simulink model "Demo_PreScanCarSim3D_cs"  (Simulink 7.6)
settings: Solver=ode5  SolverMode=SingleTasking  StartTime=0.0  StopTime=68  FixedStep=1/400  RelTol=1e-3
PreLoadFcn:
  | check_NUTS_defined;
  | 
  | assignin('base',['model_closed_' bdroot],false);
InitFcn:
  | PreScanExperimentInitFcn(bdroot)
StopFcn:
  | PreScanExperimentStopFcn(bdroot)
undefined symbols (not defined in the file or in its folder): DiscIntNeverNeededParam, warningInitialVelocity, x0, x_ini_VRML, y_ini_VRML, z_ini_VRML
libraries: PreScanSimulinkLibrary x13, simulink_extras x5, PreScanUsefulBlocks x5, simulink x3, Solver_SF x1
(part 5 of 10)

== system Demo_PreScanCarSim3D_cs/Audi_A8_1/CarSim_Vehicle ==
  note: Source model: .\CarSim_Data\Extensions\Simulink\CarSim_VehicleDynamics.mdl
  note: For state mode 'Dynamic' positions
      | are not taken into account, as they
      | are computed by integrating velocity.
      | Click annotation for Help.
  PathFollower_In : Inport
  Contact_In : Inport  Port=2
  CarSim S-Function : Solver_SF/CarSim S-Function  Priority=1  VehicleCode=i_i  SIMFILE=./CarSim_Data/simfile.sim
  CarSim2PreScanSTATE : Subsystem  mask(CarSim2PreScan:){z0=0.241}
      mask prompts: z0 "PreScan Actor initial COG z-position wrt GLOBAL axis system [m]"
      mask help: This block converts the outputs coming from the CarSim block into consistent PreScan signals.
  CarSim2PreScan_BUS : Subsystem  mask(PreScan block: CarSim to PreScan BUS){TyreRadius=0.358, cogZOffset=0.241}
      mask prompts: TyreRadius "Tyre Radius [m]"; cogZOffset "cog Z offset [m]"
      mask help: CarSim to PreScan BUS selector
      mask Help: eval('openHelp()')
      mask Display: disp('PreScan BUS\nVehicleDynamics')
  CarSim2PreScan_ContactAdapter : Subsystem  Tag=CarSim2PreScan_ContactAdapter  mask{wheelRadius=0.358}
      mask prompts: wheelRadius "Wheel radius:"
  Demux2 : Demux  Outputs=3
  Mux : Mux  Inputs=[1 1 1 12]
  MuxState : Subsystem  Tag=MuxState  mask{positioningmode=on, TimeStep=1/400}
      mask prompts: positioningmode "Positioning Mode"; TimeStep "Auto Assigned: Time Step [s]"
      settings: DeleteFcn=PreScanBlockDeleteFcn;
  TyreContact To Road Information : Subsystem  mask{Roll0=0, Pitch0=0, Yaw0=0.029771632590382069}
      mask prompts: Roll0 "Ini roll-angle BODY wrt VEHICLE axis system [deg]"; Pitch0 "Ini pitch-angle BODY wrt VEHICLE axis system [deg]"; Yaw0 "Ini yaw-angle VEHICLE wrt GLOBAL axis system [deg]"
  State : Outport
  State_BUS : Outport  Port=2
  ContactParams : Outport  Port=3
  wires:
  Mux/1 -> CarSim S-Function/1
  Demux2/1 -> Mux/1
  Demux2/2 -> Mux/2
  Demux2/3 -> Mux/3
  PathFollower_In/1 -> Demux2/1
  TyreContact To Road Information/1(RoadSlopeAndZ_[FL;FR;RL;RR]) -> Mux/4
  CarSim2PreScan_BUS/1(PreScanBUS_VehicleDynamics) -> State_BUS/1, CarSim2PreScan_ContactAdapter/2(State_Bus)
  CarSim S-Function/1 -> CarSim2PreScanSTATE/1(CarSim_In), CarSim2PreScan_BUS/1(CarSim_In)
  Contact_In/1 -> TyreContact To Road Information/1(TyreInfo_in)
  MuxState/1(state) -> State/1, CarSim2PreScan_ContactAdapter/1(State)
  CarSim2PreScan_ContactAdapter/1(ContactParams) -> ContactParams/1
  CarSim2PreScanSTATE/9(Y [rad]) -> MuxState/9(Y [rad])
  CarSim2PreScanSTATE/8(P [rad]) -> MuxState/8(P [rad])
  CarSim2PreScanSTATE/7(R [rad]) -> MuxState/7(R [rad])
  CarSim2PreScanSTATE/6(dz [m/s]) -> MuxState/6(dz [m/s])
  CarSim2PreScanSTATE/5(dy [m/s]) -> MuxState/5(dy [m/s])
  CarSim2PreScanSTATE/4(dx [m/s]) -> MuxState/4(dx [m/s])
  CarSim2PreScanSTATE/3(z [m]) -> MuxState/3(z [m])
  CarSim2PreScanSTATE/2(y [m]) -> MuxState/2(y [m])
  CarSim2PreScanSTATE/1(x [m]) -> MuxState/1(x [m])

== system Demo_PreScanCarSim3D_cs/Audi_A8_1/PathFollower_Preview_1 ==
  TrajOffset x,y,Y [m,m,deg] : Inport
  ActorOffset_Left(+) / Right(-) [m] : Inport  Port=2
  position x,y,Y [m,m,deg] : Inport  Port=3
  Initial Velocity [m/s] : Inport  Port=4
  Desired Velocity [m/s] : Inport  Port=5
  velocity [m/s] : Inport  Port=6
  vx [m/s] : Inport  Port=7
  vy [m/s] : Inport  Port=8
  Yaw rate [deg/s] : Inport  Port=9
  CorneringStiffness_Tyres_Front [N/rad] : Inport  Port=10
  CorneringStiffness_Tyres_Rear [N/rad] : Inport  Port=11
  steering_ratio[-] : Inport  Port=12
  LateralController : Subsystem
  LongitudinalController : Subsystem
  delta_steerwheel [deg] : Outport
  throttle [%] : Outport  Port=2
  brake pressure [bar] : Outport  Port=3
  v0 [m/s] : Outport  Port=4
  Auto_GearShift : Outport  Port=5
  Actor/Traj_distance [m] : Outport  Port=6
  Actor/Traj_angle [deg] : Outport  Port=7
  wires:
  LateralController/3(delta_steerwheel [deg]) -> delta_steerwheel [deg]/1
  steering_ratio[-]/1 -> LateralController/9(steering_ratio[-])
  CorneringStiffness_Tyres_Rear [N/rad]/1 -> LateralController/8(CorneringStiffness_Tyres_Rear [N/rad])
  CorneringStiffness_Tyres_Front [N/rad]/1 -> LateralController/7(CorneringStiffness_Tyres_Front [N/rad])
  Yaw rate [deg/s]/1 -> LateralController/6(Yaw rate [deg/s])
  vy [m/s]/1 -> LateralController/5(vy [m/s])
  vx [m/s]/1 -> LateralController/4(vx [m/s])
  position x,y,Y [m,m,deg]/1 -> LateralController/3(position x,y,Y [m,m,deg])
  ActorOffset_Left(+) / Right(-) [m]/1 -> LateralController/2(ActorOffset_Left(+) / Right(-) [m])
  TrajOffset x,y,Y [m,m,deg]/1 -> LateralController/1(TrajOffset x,y,Y [m,m,deg])
  LateralController/2(Actor/Traj_angle [deg]) -> Actor/Traj_angle [deg]/1
  LateralController/1(Actor/Traj_distance [m]) -> Actor/Traj_distance [m]/1
  velocity [m/s]/1 -> LongitudinalController/1(v_actual [m/s])
  LongitudinalController/1(throttle [%]) -> throttle [%]/1
  Desired Velocity [m/s]/1 -> LongitudinalController/2(Desired Velocity [m/s])
  Initial Velocity [m/s]/1 -> LongitudinalController/3(Initial Velocity [m/s])
  LongitudinalController/2(brake pressure [bar]) -> brake pressure [bar]/1
  LongitudinalController/3(v0 [m/s]) -> v0 [m/s]/1
  LongitudinalController/4(Auto_GearShift) -> Auto_GearShift/1

== system Demo_PreScanCarSim3D_cs/Audi_A8_1/PreScan_RayCast_Contact_Sensor ==
  ContactParams : Inport  SampleTime=TimeStep
  Bus Creator2 : BusCreator
  Constant : Constant  Value=0
  Contact Point Bus Creator : Subsystem
  Contact Point Bus Creator1 : Subsystem
  Contact Point Bus Creator2 : Subsystem
  Contact Point Bus Creator3 : Subsystem
  Demux : Demux
  Demux1 : Demux  Outputs=[9 1 12 4]
  Demux2 : Demux
  Level-2 M-file S-Function : M-S-Function  FunctionName=msfcn_wheelPoseCorrection  Parameters=nrOfWheels  mask{nrOfWheels=4}
      mask prompts: nrOfWheels "Number of Wheels:"
      mask Display:
      | port_label('input', 1,'Wheel poses')
      | port_label('input', 2,'Wheel radius')
      | port_label('input', 3,'Vehicle orientation')
      | 
      | port_label('output', 1,'Virtual poses')
  Level-2 MATLAB S-Function : M-S-Function  FunctionName=msfcn_wheelContacts_raycast  Parameters=NumberOfWheels, MaxContactPoints, Range  mask{NumberOfWheels=4, MaxContactPoints=1, Range=4}
      mask prompts: NumberOfWheels "Number of Wheels:"; MaxContactPoints "Maximum number of Contact Points:"; Range "Range of ray [m]:"
      mask Display:
      | port_label('input', 1, 'Wheel poses')
      | 
      | port_label('output', 1, 'Contacts')
  Level-2 MATLAB S-Function1 : M-S-Function  FunctionName=msfcn_CollisionConv  Parameters=NumberOfWheels hcog b  mask{NumberOfWheels=4}
      mask prompts: NumberOfWheels "Number of Wheels:"
      settings: AttributesFormatString=Wheels = %<NumberOfWheels>
      mask Display:
      | port_label('input', 1,'Vehicle wrt World')
      | port_label('input', 2,'Wheels wrt World')
  Mux6 : Mux  Inputs=2
  Rate Transition : RateTransition  OutPortSampleTimeOpt=Inherit
  Vehicle Local to World : Subsystem
  Wheels Local to World : Subsystem  Tag=MuxWheels
      settings: DeleteFcn=PreScanBlockDeleteFcn;
      mask Type: PreScan Mux Block:
  Results : Outport
  wires:
  Rate Transition/1 -> Results/1
  Demux1/4 -> Level-2 M-file S-Function/2
  Level-2 M-file S-Function/1 -> Level-2 MATLAB S-Function/1
  Level-2 MATLAB S-Function1/1 -> Level-2 M-file S-Function/1
  Mux6/1 -> Level-2 MATLAB S-Function1/1
  Level-2 MATLAB S-Function/1 -> Demux/1
  Demux/1 -> Contact Point Bus Creator/1(demux in)
  Demux/2 -> Contact Point Bus Creator1/1(demux in)
  Demux/3 -> Contact Point Bus Creator2/1(demux in)
  Demux/4 -> Contact Point Bus Creator3/1(demux in)
  Contact Point Bus Creator/1(bus out) -> Bus Creator2/1  "TireFL"
  Contact Point Bus Creator1/1(bus out) -> Bus Creator2/2  "TireFR"
  Contact Point Bus Creator2/1(bus out) -> Bus Creator2/3  "TireRL"
  Contact Point Bus Creator3/1(bus out) -> Bus Creator2/4  "TireRR"
  Vehicle Local to World/1(Position) -> Mux6/1
  Vehicle Local to World/2(Orientation) -> Level-2 M-file S-Function/3, Mux6/2
  Wheels Local to World/1(Wheel Poses) -> Level-2 MATLAB S-Function1/2
  Demux1/2 -> Wheels Local to World/3(Velocity [m/s])
  Demux2/1 -> Wheels Local to World/4(Disp FL [m])
  Demux2/2 -> Wheels Local to World/5(Disp FR [m])
  Demux2/3 -> Wheels Local to World/6(Disp RL [m])
  Demux2/4 -> Wheels Local to World/7(Disp RR [m])
  Constant/1 -> Wheels Local to World/2(Steer Angle Rear [deg]), Wheels Local to World/1(Steer Angle Front [deg])
  Bus Creator2/1 -> Rate Transition/1
  ContactParams/1 -> Demux1/1
  Demux1/1 -> Vehicle Local to World/1(State)
  Demux1/3 -> Demux2/1

== system Demo_PreScanCarSim3D_cs/Audi_A8_1/SELF_Demux ==
  SELF : Inport
  Demux1 : Demux  Outputs=3
  Demux2 : Demux  Outputs=3
  Demux3 : Demux  Outputs=[3 3 1 1]
  Demux4 : Demux  Outputs=3
  Gain : Gain  Gain=180/pi
  Gain1 : Gain  Gain=180/pi
  Selector : Selector  InputPortWidth=3  IndexOptions=Index vector (dialog)  Indices=[3]  OutputSizes=1
  compas converter : Subsystem
  xyz2GPS : PreScanUsefulBlocks/xyz2GPS  CoordinateCount=1  GPS_base=[0.000000 0.000000 0.000]
  x [m] : Outport
  y [m] : Outport  Port=2
  z [m] : Outport  Port=3
  rotx [deg] : Outport  Port=4
  roty [deg] : Outport  Port=5
  rotz [deg] : Outport  Port=6
  GPS lat [deg] : Outport  Port=7
  GPS long [deg] : Outport  Port=8
  GPS alt [m] : Outport  Port=9
  velocity [m/s] : Outport  Port=10
  heading [deg] : Outport  Port=11
  yaw rate [deg/s] : Outport  Port=12
  wires:
  Demux3/4 -> Gain1/1
  Gain1/1 -> yaw rate [deg/s]/1
  Demux3/3 -> velocity [m/s]/1
  compas converter/1(heading [deg]) -> heading [deg]/1
  xyz2GPS/1 -> Demux4/1
  Demux4/3 -> GPS alt [m]/1
  Demux4/2 -> GPS long [deg]/1
  Demux4/1 -> GPS lat [deg]/1
  Demux3/2 -> Gain/1, Selector/1
  Demux3/1 -> xyz2GPS/1, Demux1/1
  SELF/1 -> Demux3/1
  Demux2/3 -> rotz [deg]/1
  Demux2/2 -> roty [deg]/1
  Demux2/1 -> rotx [deg]/1
  Demux1/3 -> z [m]/1
  Demux1/2 -> y [m]/1
  Demux1/1 -> x [m]/1
  Gain/1 -> Demux2/1
  Selector/1 -> compas converter/1(rotz [rad])

== system Demo_PreScanCarSim3D_cs/Audi_A8_1/Trajectories ==
  Traj2State1 : Subsystem  Tag=Traj2State
      settings: DeleteFcn=PreScanBlockDeleteFcn;
      mask Type: PreScan Demux Block:
  Trajectory_1 : Subsystem  Tag=Trajectory  mask(PreScan Source Block: Trajectory){FileName='Trajectory_1.mat', TimeStep=20/400}
      mask prompts: TimeStep "Time Step [s]"
      mask help:
      | The Trajectory block contains the trajectories defined in the PreScan Experiment Editor. The output of the trajectory block is the (vehicle) State.
      |
      | For more information, please click Help.
      mask init:
      | [direc,name]=fileparts(get_param(bdroot, 'FileName'));
      | load([direc,'/Trajectories/',FileName])
      | trajectory=trajectory';
      | 
      | traj.time=trajectory(:,1);%[];
      | traj.signals.values=trajectory(:,2:19);
      | traj.dimensions=18;
      | traj.label='';
      | 
      | SampleTime=traj.time(2)-traj.time(1);
      settings: DeleteFcn=PreScanBlockDeleteFcn;
      mask Help: eval('openHelp(312)')
      mask Display: fprintf(FileName)
  Trajectory_1_Offset : Constant  Tag=TrajectoryOffset  Value="[0  0  0  0  0  0]"
  State : Outport  Tag=TrajOutport
  wires:
  Traj2State1/1(state) -> State/1
  Trajectory_1_Offset/1 -> Traj2State1/2(Offset)
  Trajectory_1/1(trajectory) -> Traj2State1/1(Traj Org)

== system Demo_PreScanCarSim3D_cs/Audi_A8_1/VISUWheelsCarSim_Mux ==
  StateWheels : Inport
  Bus Selector : BusSelector  OutputSignals=PreScanBUS_VehicleDynamics.Wheel.Position.Linear.Pos_FL_Wheel_CoorSys_V[x;y;z][m],PreScanBUS_VehicleDynamics.Wheel.Position.Angualr.Rot_FL_Wheel_CoorSys_V[x;y;z][deg].Angle_Camber_FL_Wheel_CoorSys_V[deg],PreScanBUS_VehicleDynamics.Wheel.Position.Angualr.Rot_FL_Wheel_CoorSys_V[x;y;z][deg].Angle_Rot_FL_Wheel[deg],PreScanBUS_VehicleDynamics.Wheel.Position.Angualr.Rot_FL_Wheel_CoorSys_V[x;y;z][deg].Angle_Toe_FL_Wheel_CoorSys_V[deg],PreScanBUS_VehicleDynamics.Wheel.Position.Linear.Pos_FR_Wheel_CoorSys_V[x;y;z][m],PreScanBUS_VehicleDynamics.Wheel.Position.Angualr.Rot_FR_Wheel_CoorSys_V[x;y;z][deg].Angle_Camber_FR_Wheel_CoorSys_V[deg],PreScanBUS_VehicleDynamics.Wheel.Position.Angualr.Rot_FR_Wheel_CoorSys_V[x;y;z][deg].Angle_Rot_FR_Wheel[deg],PreScanBUS_VehicleDynamics.Wheel.Position.Angualr.Rot_FR_Wheel_CoorSys_V[x;y;z][deg].Angle_Toe_FR_Wheel_CoorSys_V[deg],PreScanBUS_VehicleDynamics.Wheel.Position.Linear.Pos_RL_Wheel_CoorSys_V[x;y;z][m],PreScanBUS_VehicleDynamics.Wheel.Position.Angualr.Rot_RL_Wheel_CoorSys_V[x;y;z][deg].Angle_Camber_RL_Wheel_CoorSys_V[deg],PreScanBUS_VehicleDynamics.Wheel.Position.Angualr.Rot_RL_Wheel_CoorSys_V[x;y;z][deg].Angle_Rot_RL_Wheel[deg],PreScanBUS_VehicleDynamics.Wheel.Position.Angualr.Rot_RL_Wheel_CoorSys_V[x;y;z][deg].Angle_Toe_RL_Wheel_CoorSys_V[deg],PreScanBUS_VehicleDynamics.Wheel.Position.Linear.Pos_RR_Wheel_CoorSys_V[x;y;z][m],PreScanBUS_VehicleDynamics.Wheel.Position.Angualr.Rot_RR_Wheel_CoorSys_V[x;y;z][deg].Angle_Camber_RR_Wheel_CoorSys_V[deg],PreScanBUS_VehicleDynamics.Wheel.Position.Angualr.Rot_RR_Wheel_CoorSys_V[x;y;z][deg].Angle_Rot_RR_Wheel[deg],PreScanBUS_VehicleDynamics.Wheel.Position.Angualr.Rot_RR_Wheel_CoorSys_V[x;y;z][deg].Angle_Toe_RR_Wheel_CoorSys_V[deg]
  Demux{,1..3} (4 alike) : Demux  Outputs=3
  Mux{,1..4,6..8} (8 alike) : Mux  Inputs=3
  Mux5 : Mux  Inputs=[3 3 3 3 3 3 3 3]
  Wheels : Outport
  wires:
  Bus Selector/16 -> Mux3/3  "<Angle_Toe_RR_Wheel_CoorSys_V[deg]>"
  Bus Selector/15 -> Mux3/2  "<Angle_Rot_RR_Wheel[deg]>"
  Bus Selector/14 -> Mux3/1  "<Angle_Camber_RR_Wheel_CoorSys_V[deg]>"
  Bus Selector/13 -> Demux3/1  "<Pos_RR_Wheel_CoorSys_V[x;y;z][m]>"
  Demux3/3 -> Mux8/3
  Demux3/2 -> Mux8/2
  Demux3/1 -> Mux8/1
  Bus Selector/12 -> Mux2/3  "<Angle_Toe_RL_Wheel_CoorSys_V[deg]>"
  Bus Selector/11 -> Mux2/2  "<Angle_Rot_RL_Wheel[deg]>"
  Bus Selector/10 -> Mux2/1  "<Angle_Camber_RL_Wheel_CoorSys_V[deg]>"
  Bus Selector/9 -> Demux2/1  "<Pos_RL_Wheel_CoorSys_V[x;y;z][m]>"
  Demux2/3 -> Mux7/3
  Demux2/2 -> Mux7/2
  Demux2/1 -> Mux7/1
  Bus Selector/8 -> Mux1/3  "<Angle_Toe_FR_Wheel_CoorSys_V[deg]>"
  Bus Selector/7 -> Mux1/2  "<Angle_Rot_FR_Wheel[deg]>"
  Bus Selector/6 -> Mux1/1  "<Angle_Camber_FR_Wheel_CoorSys_V[deg]>"
  Bus Selector/5 -> Demux1/1  "<Pos_FR_Wheel_CoorSys_V[x;y;z][m]>"
  Demux1/3 -> Mux6/3
  Demux1/2 -> Mux6/2
  Demux1/1 -> Mux6/1
  Bus Selector/4 -> Mux/3  "<Angle_Toe_FL_Wheel_CoorSys_V[deg]>"
  Bus Selector/3 -> Mux/2  "<Angle_Rot_FL_Wheel[deg]>"
  Bus Selector/2 -> Mux/1  "<Angle_Camber_FL_Wheel_CoorSys_V[deg]>"
  Demux/3 -> Mux4/3
  Demux/2 -> Mux4/2
  Demux/1 -> Mux4/1
  Bus Selector/1 -> Demux/1  "<Pos_FL_Wheel_CoorSys_V[x;y;z][m]>"
  StateWheels/1 -> Bus Selector/1
  Mux2/1 -> Mux5/6  "xyz rotation RL [deg]"
  Mux3/1 -> Mux5/8  "xyz rotation RR [deg]"
  Mux/1 -> Mux5/2  "xyz rotation FL [deg]"
  Mux1/1 -> Mux5/4  "xyz rotation FR [deg]"
  Mux5/1 -> Wheels/1
  Mux4/1 -> Mux5/1  "xyz displacement FL [m]"
  Mux6/1 -> Mux5/3  "xyz displacement FR [m]"
  Mux8/1 -> Mux5/7  "xyz displacement RR [m]"
  Mux7/1 -> Mux5/5  "xyz displacement RL [m]"

== system Demo_PreScanCarSim3D_cs/Box_1/Dynamics_Empty ==
  note: For state mode 'Dynamic' positions
      | are not taken into account, as they
      | are computed by integrating velocity.
      | Click annotation for Help.
  Ground_{1..9} (9 alike) : Ground
  MuxState : Subsystem  Tag=MuxState  mask{positioningmode=off, TimeStep=20/400}
      mask prompts: positioningmode "Positioning Mode"; TimeStep "Auto Assigned: Time Step [s]"
      settings: DeleteFcn=PreScanBlockDeleteFcn;
  State : Outport  Tag=StateOutport
  wires:
  Ground_9/1 -> MuxState/9(Y [rad])
  Ground_8/1 -> MuxState/8(P [rad])
  Ground_7/1 -> MuxState/7(R [rad])
  Ground_6/1 -> MuxState/6(dz [m/s])
  Ground_5/1 -> MuxState/5(dy [m/s])
  Ground_4/1 -> MuxState/4(dx [m/s])
  Ground_3/1 -> MuxState/3(z [m])
  Ground_2/1 -> MuxState/2(y [m])
  Ground_1/1 -> MuxState/1(x [m])
  MuxState/1(state) -> State/1

== system Demo_PreScanCarSim3D_cs/Box_1/SELF_Demux ==
  SELF : Inport
  Demux1 : Demux  Outputs=3
  Demux2 : Demux  Outputs=3
  Demux3 : Demux  Outputs=[3 3 1 1]
  Demux4 : Demux  Outputs=3
  Gain : Gain  Gain=180/pi
  Gain1 : Gain  Gain=180/pi
  Selector : Selector  InputPortWidth=3  IndexOptions=Index vector (dialog)  Indices=[3]  OutputSizes=1
  compas converter : Subsystem
  xyz2GPS : PreScanUsefulBlocks/xyz2GPS  CoordinateCount=1  GPS_base=[0.000000 0.000000 0.000]
  x [m] : Outport
  y [m] : Outport  Port=2
  z [m] : Outport  Port=3
  rotx [deg] : Outport  Port=4
  roty [deg] : Outport  Port=5
  rotz [deg] : Outport  Port=6
  GPS lat [deg] : Outport  Port=7
  GPS long [deg] : Outport  Port=8
  GPS alt [m] : Outport  Port=9
  velocity [m/s] : Outport  Port=10
  heading [deg] : Outport  Port=11
  yaw rate [deg/s] : Outport  Port=12
  wires:
  Demux3/4 -> Gain1/1
  Gain1/1 -> yaw rate [deg/s]/1
  Demux3/3 -> velocity [m/s]/1
  compas converter/1(heading [deg]) -> heading [deg]/1
  xyz2GPS/1 -> Demux4/1
  Demux4/3 -> GPS alt [m]/1
  Demux4/2 -> GPS long [deg]/1
  Demux4/1 -> GPS lat [deg]/1
  Demux3/2 -> Gain/1, Selector/1
  Demux3/1 -> xyz2GPS/1, Demux1/1
  SELF/1 -> Demux3/1
  Demux2/3 -> rotz [deg]/1
  Demux2/2 -> roty [deg]/1
  Demux2/1 -> rotx [deg]/1
  Demux1/3 -> z [m]/1
  Demux1/2 -> y [m]/1
  Demux1/1 -> x [m]/1
  Gain/1 -> Demux2/1
  Selector/1 -> compas converter/1(rotz [rad])

== system Demo_PreScanCarSim3D_cs/Box_2/Dynamics_Empty ==
  note: For state mode 'Dynamic' positions
      | are not taken into account, as they
      | are computed by integrating velocity.
      | Click annotation for Help.
  Ground_{1..9} (9 alike) : Ground
  MuxState : Subsystem  Tag=MuxState  mask{positioningmode=off, TimeStep=20/400}
      mask prompts: positioningmode "Positioning Mode"; TimeStep "Auto Assigned: Time Step [s]"
      settings: DeleteFcn=PreScanBlockDeleteFcn;
  State : Outport  Tag=StateOutport
  wires:
  Ground_9/1 -> MuxState/9(Y [rad])
  Ground_8/1 -> MuxState/8(P [rad])
  Ground_7/1 -> MuxState/7(R [rad])
  Ground_6/1 -> MuxState/6(dz [m/s])
  Ground_5/1 -> MuxState/5(dy [m/s])
  Ground_4/1 -> MuxState/4(dx [m/s])
  Ground_3/1 -> MuxState/3(z [m])
  Ground_2/1 -> MuxState/2(y [m])
  Ground_1/1 -> MuxState/1(x [m])
  MuxState/1(state) -> State/1

== system Demo_PreScanCarSim3D_cs/Box_2/SELF_Demux ==
  SELF : Inport
  Demux1 : Demux  Outputs=3
  Demux2 : Demux  Outputs=3
  Demux3 : Demux  Outputs=[3 3 1 1]
  Demux4 : Demux  Outputs=3
  Gain : Gain  Gain=180/pi
  Gain1 : Gain  Gain=180/pi
  Selector : Selector  InputPortWidth=3  IndexOptions=Index vector (dialog)  Indices=[3]  OutputSizes=1
  compas converter : Subsystem
  xyz2GPS : PreScanUsefulBlocks/xyz2GPS  CoordinateCount=1  GPS_base=[0.000000 0.000000 0.000]
  x [m] : Outport
  y [m] : Outport  Port=2
  z [m] : Outport  Port=3
  rotx [deg] : Outport  Port=4
  roty [deg] : Outport  Port=5
  rotz [deg] : Outport  Port=6
  GPS lat [deg] : Outport  Port=7
  GPS long [deg] : Outport  Port=8
  GPS alt [m] : Outport  Port=9
  velocity [m/s] : Outport  Port=10
  heading [deg] : Outport  Port=11
  yaw rate [deg/s] : Outport  Port=12
  wires:
  Demux3/4 -> Gain1/1
  Gain1/1 -> yaw rate [deg/s]/1
  Demux3/3 -> velocity [m/s]/1
  compas converter/1(heading [deg]) -> heading [deg]/1
  xyz2GPS/1 -> Demux4/1
  Demux4/3 -> GPS alt [m]/1
  Demux4/2 -> GPS long [deg]/1
  Demux4/1 -> GPS lat [deg]/1
  Demux3/2 -> Gain/1, Selector/1
  Demux3/1 -> xyz2GPS/1, Demux1/1
  SELF/1 -> Demux3/1
  Demux2/3 -> rotz [deg]/1
  Demux2/2 -> roty [deg]/1
  Demux2/1 -> rotx [deg]/1
  Demux1/3 -> z [m]/1
  Demux1/2 -> y [m]/1
  Demux1/1 -> x [m]/1
  Gain/1 -> Demux2/1
  Selector/1 -> compas converter/1(rotz [rad])

== system Demo_PreScanCarSim3D_cs/Box_3/Dynamics_Empty ==
  note: For state mode 'Dynamic' positions
      | are not taken into account, as they
      | are computed by integrating velocity.
      | Click annotation for Help.
  Ground_{1..9} (9 alike) : Ground
  MuxState : Subsystem  Tag=MuxState  mask{positioningmode=off, TimeStep=20/400}
      mask prompts: positioningmode "Positioning Mode"; TimeStep "Auto Assigned: Time Step [s]"
      settings: DeleteFcn=PreScanBlockDeleteFcn;
  State : Outport  Tag=StateOutport
  wires:
  Ground_9/1 -> MuxState/9(Y [rad])
  Ground_8/1 -> MuxState/8(P [rad])
  Ground_7/1 -> MuxState/7(R [rad])
  Ground_6/1 -> MuxState/6(dz [m/s])
  Ground_5/1 -> MuxState/5(dy [m/s])
  Ground_4/1 -> MuxState/4(dx [m/s])
  Ground_3/1 -> MuxState/3(z [m])
  Ground_2/1 -> MuxState/2(y [m])
  Ground_1/1 -> MuxState/1(x [m])
  MuxState/1(state) -> State/1

== system Demo_PreScanCarSim3D_cs/Box_3/SELF_Demux ==
  SELF : Inport
  Demux1 : Demux  Outputs=3
  Demux2 : Demux  Outputs=3
  Demux3 : Demux  Outputs=[3 3 1 1]
  Demux4 : Demux  Outputs=3
  Gain : Gain  Gain=180/pi
  Gain1 : Gain  Gain=180/pi
  Selector : Selector  InputPortWidth=3  IndexOptions=Index vector (dialog)  Indices=[3]  OutputSizes=1
  compas converter : Subsystem
  xyz2GPS : PreScanUsefulBlocks/xyz2GPS  CoordinateCount=1  GPS_base=[0.000000 0.000000 0.000]
  x [m] : Outport
  y [m] : Outport  Port=2
  z [m] : Outport  Port=3
  rotx [deg] : Outport  Port=4
  roty [deg] : Outport  Port=5
  rotz [deg] : Outport  Port=6
  GPS lat [deg] : Outport  Port=7
  GPS long [deg] : Outport  Port=8
  GPS alt [m] : Outport  Port=9
  velocity [m/s] : Outport  Port=10
  heading [deg] : Outport  Port=11
  yaw rate [deg/s] : Outport  Port=12
  wires:
  Demux3/4 -> Gain1/1
  Gain1/1 -> yaw rate [deg/s]/1
  Demux3/3 -> velocity [m/s]/1
  compas converter/1(heading [deg]) -> heading [deg]/1
  xyz2GPS/1 -> Demux4/1
  Demux4/3 -> GPS alt [m]/1
  Demux4/2 -> GPS long [deg]/1
  Demux4/1 -> GPS lat [deg]/1
  Demux3/2 -> Gain/1, Selector/1
  Demux3/1 -> xyz2GPS/1, Demux1/1
  SELF/1 -> Demux3/1
  Demux2/3 -> rotz [deg]/1
  Demux2/2 -> roty [deg]/1
  Demux2/1 -> rotx [deg]/1
  Demux1/3 -> z [m]/1
  Demux1/2 -> y [m]/1
  Demux1/1 -> x [m]/1
  Gain/1 -> Demux2/1
  Selector/1 -> compas converter/1(rotz [rad])

== system Demo_PreScanCarSim3D_cs/Box_4/Dynamics_Empty ==
  note: For state mode 'Dynamic' positions
      | are not taken into account, as they
      | are computed by integrating velocity.
      | Click annotation for Help.
  Ground_{1..9} (9 alike) : Ground
  MuxState : Subsystem  Tag=MuxState  mask{positioningmode=off, TimeStep=20/400}
      mask prompts: positioningmode "Positioning Mode"; TimeStep "Auto Assigned: Time Step [s]"
      settings: DeleteFcn=PreScanBlockDeleteFcn;
  State : Outport  Tag=StateOutport
  wires:
  Ground_9/1 -> MuxState/9(Y [rad])
  Ground_8/1 -> MuxState/8(P [rad])
  Ground_7/1 -> MuxState/7(R [rad])
  Ground_6/1 -> MuxState/6(dz [m/s])
  Ground_5/1 -> MuxState/5(dy [m/s])
  Ground_4/1 -> MuxState/4(dx [m/s])
  Ground_3/1 -> MuxState/3(z [m])
  Ground_2/1 -> MuxState/2(y [m])
  Ground_1/1 -> MuxState/1(x [m])
  MuxState/1(state) -> State/1

== system Demo_PreScanCarSim3D_cs/Box_4/SELF_Demux ==
  SELF : Inport
  Demux1 : Demux  Outputs=3
  Demux2 : Demux  Outputs=3
  Demux3 : Demux  Outputs=[3 3 1 1]
  Demux4 : Demux  Outputs=3
  Gain : Gain  Gain=180/pi
  Gain1 : Gain  Gain=180/pi
  Selector : Selector  InputPortWidth=3  IndexOptions=Index vector (dialog)  Indices=[3]  OutputSizes=1
  compas converter : Subsystem
  xyz2GPS : PreScanUsefulBlocks/xyz2GPS  CoordinateCount=1  GPS_base=[0.000000 0.000000 0.000]
  x [m] : Outport
  y [m] : Outport  Port=2
  z [m] : Outport  Port=3
  rotx [deg] : Outport  Port=4
  roty [deg] : Outport  Port=5
  rotz [deg] : Outport  Port=6
  GPS lat [deg] : Outport  Port=7
  GPS long [deg] : Outport  Port=8
  GPS alt [m] : Outport  Port=9
  velocity [m/s] : Outport  Port=10
  heading [deg] : Outport  Port=11
  yaw rate [deg/s] : Outport  Port=12
  wires:
  Demux3/4 -> Gain1/1
  Gain1/1 -> yaw rate [deg/s]/1
  Demux3/3 -> velocity [m/s]/1
  compas converter/1(heading [deg]) -> heading [deg]/1
  xyz2GPS/1 -> Demux4/1
  Demux4/3 -> GPS alt [m]/1
  Demux4/2 -> GPS long [deg]/1
  Demux4/1 -> GPS lat [deg]/1
  Demux3/2 -> Gain/1, Selector/1
  Demux3/1 -> xyz2GPS/1, Demux1/1
  SELF/1 -> Demux3/1
  Demux2/3 -> rotz [deg]/1
  Demux2/2 -> roty [deg]/1
  Demux2/1 -> rotx [deg]/1
  Demux1/3 -> z [m]/1
  Demux1/2 -> y [m]/1
  Demux1/1 -> x [m]/1
  Gain/1 -> Demux2/1
  Selector/1 -> compas converter/1(rotz [rad])

== system Demo_PreScanCarSim3D_cs/HighwayOverhang_1/VISUMatrixSignLights_Mux ==
  MatrixSign_1 : Inport  PortDimensions=4
  MatrixSign_2 : Inport  Port=2  PortDimensions=4
  MatrixSign_3 : Inport  Port=3  PortDimensions=4
  MatrixSign_4 : Inport  Port=4  PortDimensions=4
  Saturation : Saturate  UpperLimit=1  LowerLimit=0
  SubMuxMatrixSignLights : Mux
  MatrixSignLights : Outport
  wires:
  SubMuxMatrixSignLights/1 -> Saturation/1
  MatrixSign_1/1 -> SubMuxMatrixSignLights/1
  Saturation/1 -> MatrixSignLights/1
  MatrixSign_2/1 -> SubMuxMatrixSignLights/2
  MatrixSign_3/1 -> SubMuxMatrixSignLights/3
  MatrixSign_4/1 -> SubMuxMatrixSignLights/4

== system Demo_PreScanCarSim3D_cs/HighwayOverhang_1/VISUMatrixSign_Mux ==
  MatrixSign_1 : Inport
  MatrixSign_2 : Inport  Port=2
  MatrixSign_3 : Inport  Port=3
  MatrixSign_4 : Inport  Port=4
  MatrixSign_1_InitialResource : Constant  Value=6
  MatrixSign_1_Switch : Switch  Criteria=u2 ~= 0
  MatrixSign_2_InitialResource : Constant  Value=5
  MatrixSign_2_Switch : Switch  Criteria=u2 ~= 0
  MatrixSign_3_InitialResource : Constant  Value=5
  MatrixSign_3_Switch : Switch  Criteria=u2 ~= 0
  MatrixSign_4_InitialResource : Constant  Value=5
  MatrixSign_4_Switch : Switch  Criteria=u2 ~= 0
  SubMuxMatrixSign : Mux
  MatrixSigns : Outport
  wires:
  SubMuxMatrixSign/1 -> MatrixSigns/1
  MatrixSign_1/1 -> MatrixSign_1_Switch/1, MatrixSign_1_Switch/2
  MatrixSign_1_InitialResource/1 -> MatrixSign_1_Switch/3
  MatrixSign_1_Switch/1 -> SubMuxMatrixSign/1
  MatrixSign_2/1 -> MatrixSign_2_Switch/1, MatrixSign_2_Switch/2
  MatrixSign_2_InitialResource/1 -> MatrixSign_2_Switch/3
  MatrixSign_2_Switch/1 -> SubMuxMatrixSign/2
  MatrixSign_3/1 -> MatrixSign_3_Switch/1, MatrixSign_3_Switch/2
  MatrixSign_3_InitialResource/1 -> MatrixSign_3_Switch/3
  MatrixSign_3_Switch/1 -> SubMuxMatrixSign/3
  MatrixSign_4/1 -> MatrixSign_4_Switch/1, MatrixSign_4_Switch/2
  MatrixSign_4_InitialResource/1 -> MatrixSign_4_Switch/3
  MatrixSign_4_Switch/1 -> SubMuxMatrixSign/4

== system Demo_PreScanCarSim3D_cs/HighwayOverhang_2/VISUMatrixSignLights_Mux ==
  MatrixSign_5 : Inport  PortDimensions=4
  MatrixSign_6 : Inport  Port=2  PortDimensions=4
  MatrixSign_7 : Inport  Port=3  PortDimensions=4
  Saturation : Saturate  UpperLimit=1  LowerLimit=0
  SubMuxMatrixSignLights : Mux  Inputs=3
  MatrixSignLights : Outport
  wires:
  SubMuxMatrixSignLights/1 -> Saturation/1
  MatrixSign_5/1 -> SubMuxMatrixSignLights/1
  Saturation/1 -> MatrixSignLights/1
  MatrixSign_6/1 -> SubMuxMatrixSignLights/2
  MatrixSign_7/1 -> SubMuxMatrixSignLights/3

== system Demo_PreScanCarSim3D_cs/HighwayOverhang_2/VISUMatrixSign_Mux ==
  MatrixSign_5 : Inport
  MatrixSign_6 : Inport  Port=2
  MatrixSign_7 : Inport  Port=3
  MatrixSign_5_InitialResource : Constant  Value=5
  MatrixSign_5_Switch : Switch  Criteria=u2 ~= 0
  MatrixSign_6_InitialResource : Constant  Value=5
  MatrixSign_6_Switch : Switch  Criteria=u2 ~= 0
  MatrixSign_7_InitialResource : Constant  Value=5
  MatrixSign_7_Switch : Switch  Criteria=u2 ~= 0
  SubMuxMatrixSign : Mux  Inputs=3
  MatrixSigns : Outport
  wires:
  SubMuxMatrixSign/1 -> MatrixSigns/1
  MatrixSign_5/1 -> MatrixSign_5_Switch/1, MatrixSign_5_Switch/2
  MatrixSign_5_InitialResource/1 -> MatrixSign_5_Switch/3
  MatrixSign_5_Switch/1 -> SubMuxMatrixSign/1
  MatrixSign_6/1 -> MatrixSign_6_Switch/1, MatrixSign_6_Switch/2
  MatrixSign_6_InitialResource/1 -> MatrixSign_6_Switch/3
  MatrixSign_6_Switch/1 -> SubMuxMatrixSign/2
  MatrixSign_7/1 -> MatrixSign_7_Switch/1, MatrixSign_7_Switch/2
  MatrixSign_7_InitialResource/1 -> MatrixSign_7_Switch/3
  MatrixSign_7_Switch/1 -> SubMuxMatrixSign/3

== system Demo_PreScanCarSim3D_cs/HighwayOverhang_3/VISUMatrixSignLights_Mux ==
  MatrixSign_10 : Inport  PortDimensions=4
  MatrixSign_11 : Inport  Port=2  PortDimensions=4
  MatrixSign_12 : Inport  Port=3  PortDimensions=4
  Saturation : Saturate  UpperLimit=1  LowerLimit=0
  SubMuxMatrixSignLights : Mux  Inputs=3
  MatrixSignLights : Outport
  wires:
  SubMuxMatrixSignLights/1 -> Saturation/1
  MatrixSign_10/1 -> SubMuxMatrixSignLights/1
  Saturation/1 -> MatrixSignLights/1
  MatrixSign_11/1 -> SubMuxMatrixSignLights/2
  MatrixSign_12/1 -> SubMuxMatrixSignLights/3

== system Demo_PreScanCarSim3D_cs/HighwayOverhang_3/VISUMatrixSign_Mux ==
  MatrixSign_10 : Inport
  MatrixSign_11 : Inport  Port=2
  MatrixSign_12 : Inport  Port=3
  MatrixSign_10_InitialResource : Constant  Value=9
  MatrixSign_10_Switch : Switch  Criteria=u2 ~= 0
  MatrixSign_11_InitialResource : Constant  Value=9
  MatrixSign_11_Switch : Switch  Criteria=u2 ~= 0
  MatrixSign_12_InitialResource : Constant  Value=9
  MatrixSign_12_Switch : Switch  Criteria=u2 ~= 0
  SubMuxMatrixSign : Mux  Inputs=3
  MatrixSigns : Outport
  wires:
  SubMuxMatrixSign/1 -> MatrixSigns/1
  MatrixSign_10/1 -> MatrixSign_10_Switch/1, MatrixSign_10_Switch/2
  MatrixSign_10_InitialResource/1 -> MatrixSign_10_Switch/3
  MatrixSign_10_Switch/1 -> SubMuxMatrixSign/1
  MatrixSign_11/1 -> MatrixSign_11_Switch/1, MatrixSign_11_Switch/2
  MatrixSign_11_InitialResource/1 -> MatrixSign_11_Switch/3
  MatrixSign_11_Switch/1 -> SubMuxMatrixSign/2
  MatrixSign_12/1 -> MatrixSign_12_Switch/1, MatrixSign_12_Switch/2
  MatrixSign_12_InitialResource/1 -> MatrixSign_12_Switch/3
  MatrixSign_12_Switch/1 -> SubMuxMatrixSign/3

== system Demo_PreScanCarSim3D_cs/HighwayOverhang_5/VISUMatrixSignLights_Mux ==
  MatrixSign_18 : Inport  PortDimensions=4
  MatrixSign_19 : Inport  Port=2  PortDimensions=4
  MatrixSign_20 : Inport  Port=3  PortDimensions=4
  Saturation : Saturate  UpperLimit=1  LowerLimit=0
  SubMuxMatrixSignLights : Mux  Inputs=3
  MatrixSignLights : Outport
  wires:
  SubMuxMatrixSignLights/1 -> Saturation/1
  MatrixSign_18/1 -> SubMuxMatrixSignLights/1
  Saturation/1 -> MatrixSignLights/1
  MatrixSign_19/1 -> SubMuxMatrixSignLights/2
  MatrixSign_20/1 -> SubMuxMatrixSignLights/3

== system Demo_PreScanCarSim3D_cs/HighwayOverhang_5/VISUMatrixSign_Mux ==
  MatrixSign_18 : Inport
  MatrixSign_19 : Inport  Port=2
  MatrixSign_20 : Inport  Port=3
  MatrixSign_18_InitialResource : Constant  Value=11
  MatrixSign_18_Switch : Switch  Criteria=u2 ~= 0
  MatrixSign_19_InitialResource : Constant  Value=11
  MatrixSign_19_Switch : Switch  Criteria=u2 ~= 0
  MatrixSign_20_InitialResource : Constant  Value=11
  MatrixSign_20_Switch : Switch  Criteria=u2 ~= 0
  SubMuxMatrixSign : Mux  Inputs=3
  MatrixSigns : Outport
  wires:
  SubMuxMatrixSign/1 -> MatrixSigns/1
  MatrixSign_18/1 -> MatrixSign_18_Switch/1, MatrixSign_18_Switch/2
  MatrixSign_18_InitialResource/1 -> MatrixSign_18_Switch/3
  MatrixSign_18_Switch/1 -> SubMuxMatrixSign/1
  MatrixSign_19/1 -> MatrixSign_19_Switch/1, MatrixSign_19_Switch/2
  MatrixSign_19_InitialResource/1 -> MatrixSign_19_Switch/3
  MatrixSign_19_Switch/1 -> SubMuxMatrixSign/2
  MatrixSign_20/1 -> MatrixSign_20_Switch/1, MatrixSign_20_Switch/2
  MatrixSign_20_InitialResource/1 -> MatrixSign_20_Switch/3
  MatrixSign_20_Switch/1 -> SubMuxMatrixSign/3

== system Demo_PreScanCarSim3D_cs/STATE_Audi_A8_1/Acceleration ==
  Y : Inport
  Assignment : Assignment  IndexMode=Zero-based  SampleTime=TimeStep  IndexOptions=Starting index (dialog)  Indices=PortIndex  OutputSizes=[1 1]
  Data Store Read : DataStoreRead  DataStoreName=SimCoreActuators  SampleTime=TimeStep
  Data Store Write : DataStoreWrite  DataStoreName=SimCoreActuators
  wires:
  Assignment/1 -> Data Store Write/1
  Data Store Read/1 -> Assignment/1
  Y/1 -> Assignment/2

== system Demo_PreScanCarSim3D_cs/STATE_Audi_A8_1/Position ==
  Y : Inport
  Assignment : Assignment  IndexMode=Zero-based  SampleTime=TimeStep  IndexOptions=Starting index (dialog)  Indices=PortIndex  OutputSizes=[1 1]
  Data Store Read : DataStoreRead  DataStoreName=SimCoreActuators  SampleTime=TimeStep
  Data Store Write : DataStoreWrite  DataStoreName=SimCoreActuators
  wires:
  Y/1 -> Assignment/2
  Data Store Read/1 -> Assignment/1
  Assignment/1 -> Data Store Write/1

== system Demo_PreScanCarSim3D_cs/STATE_Audi_A8_1/RPY ==
  Y : Inport
  Assignment : Assignment  IndexMode=Zero-based  SampleTime=TimeStep  IndexOptions=Starting index (dialog)  Indices=PortIndex  OutputSizes=[1 1]
  Data Store Read : DataStoreRead  DataStoreName=SimCoreActuators  SampleTime=TimeStep
  Data Store Write : DataStoreWrite  DataStoreName=SimCoreActuators
  wires:
  Assignment/1 -> Data Store Write/1
  Data Store Read/1 -> Assignment/1
  Y/1 -> Assignment/2

== system Demo_PreScanCarSim3D_cs/STATE_Audi_A8_1/Velocity ==
  Y : Inport
  Assignment : Assignment  IndexMode=Zero-based  SampleTime=TimeStep  IndexOptions=Starting index (dialog)  Indices=PortIndex  OutputSizes=[1 1]
  Data Store Read : DataStoreRead  DataStoreName=SimCoreActuators  SampleTime=TimeStep
  Data Store Write : DataStoreWrite  DataStoreName=SimCoreActuators
  wires:
  Assignment/1 -> Data Store Write/1
  Data Store Read/1 -> Assignment/1
  Y/1 -> Assignment/2

== system Demo_PreScanCarSim3D_cs/STATE_Audi_A8_1/velRPY ==
  Y : Inport
  Assignment : Assignment  IndexMode=Zero-based  SampleTime=TimeStep  IndexOptions=Starting index (dialog)  Indices=PortIndex  OutputSizes=[1 1]
  Data Store Read : DataStoreRead  DataStoreName=SimCoreActuators  SampleTime=TimeStep
  Data Store Write : DataStoreWrite  DataStoreName=SimCoreActuators
  wires:
  Assignment/1 -> Data Store Write/1
  Data Store Read/1 -> Assignment/1
  Y/1 -> Assignment/2

== system Demo_PreScanCarSim3D_cs/STATE_Box_1/Acceleration ==
  Y : Inport
  Assignment : Assignment  IndexMode=Zero-based  SampleTime=TimeStep  IndexOptions=Starting index (dialog)  Indices=PortIndex  OutputSizes=[1 1]
  Data Store Read : DataStoreRead  DataStoreName=SimCoreActuators  SampleTime=TimeStep
  Data Store Write : DataStoreWrite  DataStoreName=SimCoreActuators
  wires:
  Assignment/1 -> Data Store Write/1
  Data Store Read/1 -> Assignment/1
  Y/1 -> Assignment/2

== system Demo_PreScanCarSim3D_cs/STATE_Box_1/Position ==
  Y : Inport
  Assignment : Assignment  IndexMode=Zero-based  SampleTime=TimeStep  IndexOptions=Starting index (dialog)  Indices=PortIndex  OutputSizes=[1 1]
  Data Store Read : DataStoreRead  DataStoreName=SimCoreActuators  SampleTime=TimeStep
  Data Store Write : DataStoreWrite  DataStoreName=SimCoreActuators
  wires:
  Y/1 -> Assignment/2
  Data Store Read/1 -> Assignment/1
  Assignment/1 -> Data Store Write/1

== system Demo_PreScanCarSim3D_cs/STATE_Box_1/RPY ==
  Y : Inport
  Assignment : Assignment  IndexMode=Zero-based  SampleTime=TimeStep  IndexOptions=Starting index (dialog)  Indices=PortIndex  OutputSizes=[1 1]
  Data Store Read : DataStoreRead  DataStoreName=SimCoreActuators  SampleTime=TimeStep
  Data Store Write : DataStoreWrite  DataStoreName=SimCoreActuators
  wires:
  Assignment/1 -> Data Store Write/1
  Data Store Read/1 -> Assignment/1
  Y/1 -> Assignment/2

== system Demo_PreScanCarSim3D_cs/STATE_Box_1/Velocity ==
  Y : Inport
  Assignment : Assignment  IndexMode=Zero-based  SampleTime=TimeStep  IndexOptions=Starting index (dialog)  Indices=PortIndex  OutputSizes=[1 1]
  Data Store Read : DataStoreRead  DataStoreName=SimCoreActuators  SampleTime=TimeStep
  Data Store Write : DataStoreWrite  DataStoreName=SimCoreActuators
  wires:
  Assignment/1 -> Data Store Write/1
  Data Store Read/1 -> Assignment/1
  Y/1 -> Assignment/2

== system Demo_PreScanCarSim3D_cs/STATE_Box_1/velRPY ==
  Y : Inport
  Assignment : Assignment  IndexMode=Zero-based  SampleTime=TimeStep  IndexOptions=Starting index (dialog)  Indices=PortIndex  OutputSizes=[1 1]
  Data Store Read : DataStoreRead  DataStoreName=SimCoreActuators  SampleTime=TimeStep
  Data Store Write : DataStoreWrite  DataStoreName=SimCoreActuators
  wires:
  Assignment/1 -> Data Store Write/1
  Data Store Read/1 -> Assignment/1
  Y/1 -> Assignment/2

== system Demo_PreScanCarSim3D_cs/STATE_Box_2/Acceleration ==
  Y : Inport
  Assignment : Assignment  IndexMode=Zero-based  SampleTime=TimeStep  IndexOptions=Starting index (dialog)  Indices=PortIndex  OutputSizes=[1 1]
  Data Store Read : DataStoreRead  DataStoreName=SimCoreActuators  SampleTime=TimeStep
  Data Store Write : DataStoreWrite  DataStoreName=SimCoreActuators
  wires:
  Assignment/1 -> Data Store Write/1
  Data Store Read/1 -> Assignment/1
  Y/1 -> Assignment/2

== system Demo_PreScanCarSim3D_cs/STATE_Box_2/Position ==
  Y : Inport
  Assignment : Assignment  IndexMode=Zero-based  SampleTime=TimeStep  IndexOptions=Starting index (dialog)  Indices=PortIndex  OutputSizes=[1 1]
  Data Store Read : DataStoreRead  DataStoreName=SimCoreActuators  SampleTime=TimeStep
  Data Store Write : DataStoreWrite  DataStoreName=SimCoreActuators
  wires:
  Y/1 -> Assignment/2
  Data Store Read/1 -> Assignment/1
  Assignment/1 -> Data Store Write/1

== system Demo_PreScanCarSim3D_cs/STATE_Box_2/RPY ==
  Y : Inport
  Assignment : Assignment  IndexMode=Zero-based  SampleTime=TimeStep  IndexOptions=Starting index (dialog)  Indices=PortIndex  OutputSizes=[1 1]
  Data Store Read : DataStoreRead  DataStoreName=SimCoreActuators  SampleTime=TimeStep
  Data Store Write : DataStoreWrite  DataStoreName=SimCoreActuators
  wires:
  Assignment/1 -> Data Store Write/1
  Data Store Read/1 -> Assignment/1
  Y/1 -> Assignment/2

== system Demo_PreScanCarSim3D_cs/STATE_Box_2/Velocity ==
  Y : Inport
  Assignment : Assignment  IndexMode=Zero-based  SampleTime=TimeStep  IndexOptions=Starting index (dialog)  Indices=PortIndex  OutputSizes=[1 1]
  Data Store Read : DataStoreRead  DataStoreName=SimCoreActuators  SampleTime=TimeStep
  Data Store Write : DataStoreWrite  DataStoreName=SimCoreActuators
  wires:
  Assignment/1 -> Data Store Write/1
  Data Store Read/1 -> Assignment/1
  Y/1 -> Assignment/2

== system Demo_PreScanCarSim3D_cs/STATE_Box_2/velRPY ==
  Y : Inport
  Assignment : Assignment  IndexMode=Zero-based  SampleTime=TimeStep  IndexOptions=Starting index (dialog)  Indices=PortIndex  OutputSizes=[1 1]
  Data Store Read : DataStoreRead  DataStoreName=SimCoreActuators  SampleTime=TimeStep
  Data Store Write : DataStoreWrite  DataStoreName=SimCoreActuators
  wires:
  Assignment/1 -> Data Store Write/1
  Data Store Read/1 -> Assignment/1
  Y/1 -> Assignment/2

== system Demo_PreScanCarSim3D_cs/STATE_Box_3/Acceleration ==
  Y : Inport
  Assignment : Assignment  IndexMode=Zero-based  SampleTime=TimeStep  IndexOptions=Starting index (dialog)  Indices=PortIndex  OutputSizes=[1 1]
  Data Store Read : DataStoreRead  DataStoreName=SimCoreActuators  SampleTime=TimeStep
  Data Store Write : DataStoreWrite  DataStoreName=SimCoreActuators
  wires:
  Assignment/1 -> Data Store Write/1
  Data Store Read/1 -> Assignment/1
  Y/1 -> Assignment/2

== system Demo_PreScanCarSim3D_cs/STATE_Box_3/Position ==
  Y : Inport
  Assignment : Assignment  IndexMode=Zero-based  SampleTime=TimeStep  IndexOptions=Starting index (dialog)  Indices=PortIndex  OutputSizes=[1 1]
  Data Store Read : DataStoreRead  DataStoreName=SimCoreActuators  SampleTime=TimeStep
  Data Store Write : DataStoreWrite  DataStoreName=SimCoreActuators
  wires:
  Y/1 -> Assignment/2
  Data Store Read/1 -> Assignment/1
  Assignment/1 -> Data Store Write/1

== system Demo_PreScanCarSim3D_cs/STATE_Box_3/RPY ==
  Y : Inport
  Assignment : Assignment  IndexMode=Zero-based  SampleTime=TimeStep  IndexOptions=Starting index (dialog)  Indices=PortIndex  OutputSizes=[1 1]
  Data Store Read : DataStoreRead  DataStoreName=SimCoreActuators  SampleTime=TimeStep
  Data Store Write : DataStoreWrite  DataStoreName=SimCoreActuators
  wires:
  Assignment/1 -> Data Store Write/1
  Data Store Read/1 -> Assignment/1
  Y/1 -> Assignment/2

== system Demo_PreScanCarSim3D_cs/STATE_Box_3/Velocity ==
  Y : Inport
  Assignment : Assignment  IndexMode=Zero-based  SampleTime=TimeStep  IndexOptions=Starting index (dialog)  Indices=PortIndex  OutputSizes=[1 1]
  Data Store Read : DataStoreRead  DataStoreName=SimCoreActuators  SampleTime=TimeStep
  Data Store Write : DataStoreWrite  DataStoreName=SimCoreActuators
  wires:
  Assignment/1 -> Data Store Write/1
  Data Store Read/1 -> Assignment/1
  Y/1 -> Assignment/2

== system Demo_PreScanCarSim3D_cs/STATE_Box_3/velRPY ==
  Y : Inport
  Assignment : Assignment  IndexMode=Zero-based  SampleTime=TimeStep  IndexOptions=Starting index (dialog)  Indices=PortIndex  OutputSizes=[1 1]
  Data Store Read : DataStoreRead  DataStoreName=SimCoreActuators  SampleTime=TimeStep
  Data Store Write : DataStoreWrite  DataStoreName=SimCoreActuators
  wires:
  Assignment/1 -> Data Store Write/1
  Data Store Read/1 -> Assignment/1
  Y/1 -> Assignment/2

== system Demo_PreScanCarSim3D_cs/STATE_Box_4/Acceleration ==
  Y : Inport
  Assignment : Assignment  IndexMode=Zero-based  SampleTime=TimeStep  IndexOptions=Starting index (dialog)  Indices=PortIndex  OutputSizes=[1 1]
  Data Store Read : DataStoreRead  DataStoreName=SimCoreActuators  SampleTime=TimeStep
  Data Store Write : DataStoreWrite  DataStoreName=SimCoreActuators
  wires:
  Assignment/1 -> Data Store Write/1
  Data Store Read/1 -> Assignment/1
  Y/1 -> Assignment/2

== system Demo_PreScanCarSim3D_cs/STATE_Box_4/Position ==
  Y : Inport
  Assignment : Assignment  IndexMode=Zero-based  SampleTime=TimeStep  IndexOptions=Starting index (dialog)  Indices=PortIndex  OutputSizes=[1 1]
  Data Store Read : DataStoreRead  DataStoreName=SimCoreActuators  SampleTime=TimeStep
  Data Store Write : DataStoreWrite  DataStoreName=SimCoreActuators
  wires:
  Y/1 -> Assignment/2
  Data Store Read/1 -> Assignment/1
  Assignment/1 -> Data Store Write/1

== system Demo_PreScanCarSim3D_cs/STATE_Box_4/RPY ==
  Y : Inport
  Assignment : Assignment  IndexMode=Zero-based  SampleTime=TimeStep  IndexOptions=Starting index (dialog)  Indices=PortIndex  OutputSizes=[1 1]
  Data Store Read : DataStoreRead  DataStoreName=SimCoreActuators  SampleTime=TimeStep
  Data Store Write : DataStoreWrite  DataStoreName=SimCoreActuators
  wires:
  Assignment/1 -> Data Store Write/1
  Data Store Read/1 -> Assignment/1
  Y/1 -> Assignment/2

== system Demo_PreScanCarSim3D_cs/STATE_Box_4/Velocity ==
  Y : Inport
  Assignment : Assignment  IndexMode=Zero-based  SampleTime=TimeStep  IndexOptions=Starting index (dialog)  Indices=PortIndex  OutputSizes=[1 1]
  Data Store Read : DataStoreRead  DataStoreName=SimCoreActuators  SampleTime=TimeStep
  Data Store Write : DataStoreWrite  DataStoreName=SimCoreActuators
  wires:
  Assignment/1 -> Data Store Write/1
  Data Store Read/1 -> Assignment/1
  Y/1 -> Assignment/2

== system Demo_PreScanCarSim3D_cs/STATE_Box_4/velRPY ==
  Y : Inport
  Assignment : Assignment  IndexMode=Zero-based  SampleTime=TimeStep  IndexOptions=Starting index (dialog)  Indices=PortIndex  OutputSizes=[1 1]
  Data Store Read : DataStoreRead  DataStoreName=SimCoreActuators  SampleTime=TimeStep
  Data Store Write : DataStoreWrite  DataStoreName=SimCoreActuators
  wires:
  Assignment/1 -> Data Store Write/1
  Data Store Read/1 -> Assignment/1
  Y/1 -> Assignment/2

== system Demo_PreScanCarSim3D_cs/TrafficLightRoadSideNL_1/VISUCasingLights_Mux ==
  Red [-] : Inport
  Orange [-] : Inport  Port=2
  Green [-] : Inport  Port=3
  Mux1 : Mux  Inputs=3
  CasingLights : Outport
  wires:
  Green [-]/1 -> Mux1/3
  Mux1/1 -> CasingLights/1
  Orange [-]/1 -> Mux1/2
  Red [-]/1 -> Mux1/1

== system Demo_PreScanCarSim3D_cs/TrafficLightRoadSideNL_2/VISUCasingLights_Mux ==
  Red [-] : Inport
  Orange [-] : Inport  Port=2
  Green [-] : Inport  Port=3
  Mux1 : Mux  Inputs=3
  CasingLights : Outport
  wires:
  Green [-]/1 -> Mux1/3
  Mux1/1 -> CasingLights/1
  Orange [-]/1 -> Mux1/2
  Red [-]/1 -> Mux1/1

== system Demo_PreScanCarSim3D_cs/TrafficLightRoadSideNL_3/VISUCasingLights_Mux ==
  Red [-] : Inport
  Orange [-] : Inport  Port=2
  Green [-] : Inport  Port=3
  Mux1 : Mux  Inputs=3
  CasingLights : Outport
  wires:
  Green [-]/1 -> Mux1/3
  Mux1/1 -> CasingLights/1
  Orange [-]/1 -> Mux1/2
  Red [-]/1 -> Mux1/1

== system Demo_PreScanCarSim3D_cs/TrafficLightRoadSideNL_5/VISUCasingLights_Mux ==
  Red [-] : Inport
  Orange [-] : Inport  Port=2
  Green [-] : Inport  Port=3
  Mux1 : Mux  Inputs=3
  CasingLights : Outport
  wires:
  Green [-]/1 -> Mux1/3
  Mux1/1 -> CasingLights/1
  Orange [-]/1 -> Mux1/2
  Red [-]/1 -> Mux1/1

== system Demo_PreScanCarSim3D_cs/TrafficLightRoadSideNL_6/VISUCasingLights_Mux ==
  Red [-] : Inport
  Orange [-] : Inport  Port=2
  Green [-] : Inport  Port=3
  Mux1 : Mux  Inputs=3
  CasingLights : Outport
  wires:
  Green [-]/1 -> Mux1/3
  Mux1/1 -> CasingLights/1
  Orange [-]/1 -> Mux1/2
  Red [-]/1 -> Mux1/1

== system Demo_PreScanCarSim3D_cs/TrafficLightRoadSideNL_7/VISUCasingLights_Mux ==
  Red [-] : Inport
  Orange [-] : Inport  Port=2
  Green [-] : Inport  Port=3
  Mux1 : Mux  Inputs=3
  CasingLights : Outport
  wires:
  Green [-]/1 -> Mux1/3
  Mux1/1 -> CasingLights/1
  Orange [-]/1 -> Mux1/2
  Red [-]/1 -> Mux1/1

== system Demo_PreScanCarSim3D_cs/VISUCasingLights_TrafficLightRoadSideNL_1/conv_Green ==
  on_off : Inport
  Constant5 : Constant  Value=[5 32 25 255 0 64 50 255 0 64 50 255 0 0 0 255]
  Constant9 : Constant  Value="[0 45 34 255  0 45 34 255  0 45 34 255  30 306 240 255]"
  Switch2 : Switch  Threshold=0.5
  RGBcolor : Outport
  wires:
  Switch2/1 -> RGBcolor/1
  on_off/1 -> Switch2/2
  Constant5/1 -> Switch2/3  "off"
  Constant9/1 -> Switch2/1  "on"

== system Demo_PreScanCarSim3D_cs/VISUCasingLights_TrafficLightRoadSideNL_1/conv_Orange ==
  on_off : Inport
  Constant2 : Constant  Value="[45 34 0 255  45 34 0 255  45 34 0 255  306 229 5 255]"
  Constant20 : Constant  Value=[32 25 5 255 64 48 5 255 64 54 5 255 0 0 0 255]
  Switch1 : Switch  Threshold=0.5
  RGBcolor : Outport
  wires:
  Constant20/1 -> Switch1/3  "off"
  Constant2/1 -> Switch1/1  "on"
  on_off/1 -> Switch1/2
  Switch1/1 -> RGBcolor/1

== system Demo_PreScanCarSim3D_cs/VISUCasingLights_TrafficLightRoadSideNL_1/conv_Red ==
  on_off : Inport
  Constant2 : Constant  Value="[45 0 0 255  45 0 0 255  45 0 0 255 306 30 30 255]"
  Constant20 : Constant  Value=[32 5 5 255 64 5 5 255 64 5 5 255 0 0 0 255]
  Switch1 : Switch  Threshold=0.5
  RGBcolor : Outport
  wires:
  Constant20/1 -> Switch1/3  "off"
  Constant2/1 -> Switch1/1  "on"
  on_off/1 -> Switch1/2
  Switch1/1 -> RGBcolor/1

== system Demo_PreScanCarSim3D_cs/VISUCasingLights_TrafficLightRoadSideNL_1/visu_CasingGreen ==
  Y : Inport
  Assignment : Assignment  IndexMode=Zero-based  SampleTime=TimeStep  IndexOptions=Starting index (dialog)  Indices=PortIndex  OutputSizes=[1 1]
  Data Store Read : DataStoreRead  DataStoreName=SimCoreActuators  SampleTime=TimeStep
  Data Store Write : DataStoreWrite  DataStoreName=SimCoreActuators
  wires:
  Assignment/1 -> Data Store Write/1
  Data Store Read/1 -> Assignment/1
  Y/1 -> Assignment/2

== system Demo_PreScanCarSim3D_cs/VISUCasingLights_TrafficLightRoadSideNL_1/visu_CasingOrange ==
  Y : Inport
  Assignment : Assignment  IndexMode=Zero-based  SampleTime=TimeStep  IndexOptions=Starting index (dialog)  Indices=PortIndex  OutputSizes=[1 1]
  Data Store Read : DataStoreRead  DataStoreName=SimCoreActuators  SampleTime=TimeStep
  Data Store Write : DataStoreWrite  DataStoreName=SimCoreActuators
  wires:
  Assignment/1 -> Data Store Write/1
  Data Store Read/1 -> Assignment/1
  Y/1 -> Assignment/2

== system Demo_PreScanCarSim3D_cs/VISUCasingLights_TrafficLightRoadSideNL_1/visu_CasingRed ==
  Y : Inport
  Assignment : Assignment  IndexMode=Zero-based  SampleTime=TimeStep  IndexOptions=Starting index (dialog)  Indices=PortIndex  OutputSizes=[1 1]
  Data Store Read : DataStoreRead  DataStoreName=SimCoreActuators  SampleTime=TimeStep
  Data Store Write : DataStoreWrite  DataStoreName=SimCoreActuators
  wires:
  Assignment/1 -> Data Store Write/1
  Data Store Read/1 -> Assignment/1
  Y/1 -> Assignment/2
